simulink model "ZeroCross_Simple"  (R2020a)
settings: Solver=FixedStepAuto  StartTime=0.0  StopTime=10.0  FixedStep=Ts_SIM  RelTol=1e-3
undefined symbols (not defined in the file): Ts_MCI_ZC
libraries: simulink x1
settings Model: Creator=BEDNASA  LastModifiedBy=BEDNASA

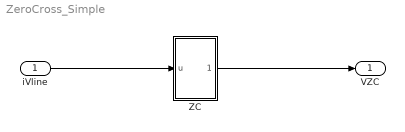
== system ZeroCross_Simple ==
  iVline : Inport
  ZC : Subsystem  TreatAsAtomicUnit=on  SystemSampleTime=Ts_MCI_ZC
  VZC : Outport
  wires:
  iVline/1 -> ZC/1(u)
  ZC/1(Out1) -> VZC/1

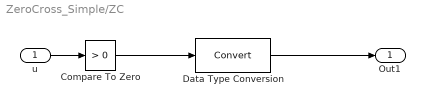
== system ZeroCross_Simple/ZC ==
  u : Inport
  Compare To Zero : simulink/Logic and Bit Operations/Compare To Zero  relop=>  OutDataTypeStr=boolean
  Data Type Conversion : DataTypeConversion
  Out1 : Outport
  wires:
  Compare To Zero/1 -> Data Type Conversion/1
  Data Type Conversion/1 -> Out1/1
  u/1 -> Compare To Zero/1
